simulink model "clarke"  (R2022b)
settings: Solver=VariableStepAuto  StartTime=0.0  StopTime=0.001  RelTol=1e-3
settings Model: Creator=15403  LastModifiedBy=15403

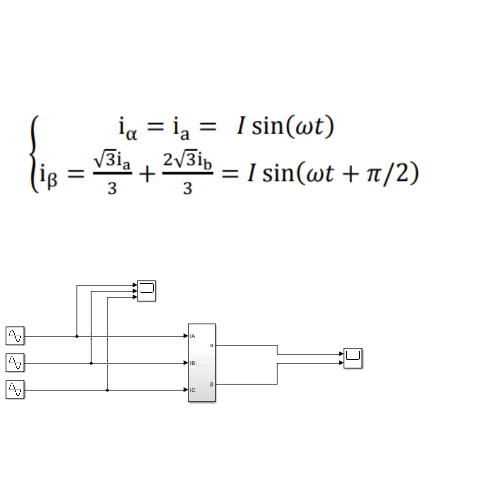
[thumbnail: Simulink's stored preview of the top-level diagram]
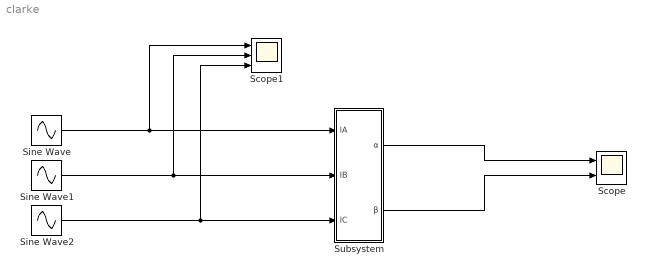
== system clarke ==
  Scope : Scope  NumInputPorts=2
  Scope1 : Scope  NumInputPorts=3
  Sine Wave : Sin  Amplitude=24/sqrt(3)  Frequency=2*pi*15000  SampleTime=0
  Sine Wave1 : Sin  Amplitude=24/sqrt(3)  Frequency=2*pi*15000  Phase=2*pi/3  SampleTime=0
  Sine Wave2 : Sin  Amplitude=24/sqrt(3)  Frequency=2*pi*15000  Phase=4*pi/3  SampleTime=0
  Subsystem : Subsystem
  wires:
  Sine Wave/1 -> Scope1/1, Subsystem/1(IA)
  Sine Wave1/1 -> Scope1/2, Subsystem/2(IB)
  Sine Wave2/1 -> Scope1/3, Subsystem/3(IC)
  Subsystem/1(α) -> Scope/1
  Subsystem/2(β) -> Scope/2

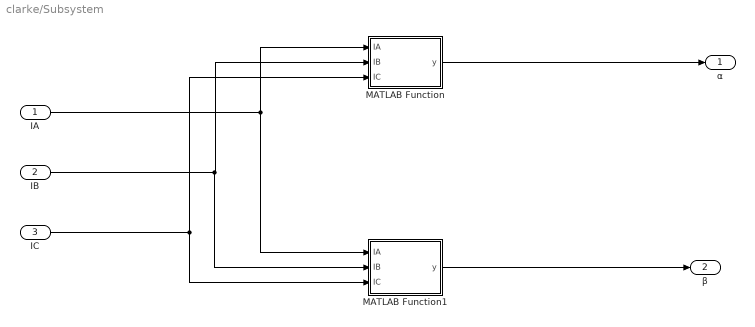
== system clarke/Subsystem ==
  IA : Inport
  IB : Inport  Port=2
  IC : Inport  Port=3
  MATLAB Function : MATLAB Function  TreatAsAtomicUnit=on
  MATLAB Function1 : MATLAB Function  TreatAsAtomicUnit=on
  α : Outport
  β : Outport  Port=2
  wires:
  MATLAB Function1/1(y) -> β/1
  MATLAB Function/1(y) -> α/1
  IA/1 -> MATLAB Function1/1(IA), MATLAB Function/1(IA)
  IB/1 -> MATLAB Function1/2(IB), MATLAB Function/2(IB)
  IC/1 -> MATLAB Function/3(IC), MATLAB Function1/3(IC)

== matlab function clarke/Subsystem/MATLAB Function1 ==
  data: IA input; y output; IB input; IC input
function y = fcn(IA, IB, IC)
%y = sqrt(3)/2 * IB - sqrt(3)/2 * IC;
y = (IB - IC) * cosd(30);

== matlab function clarke/Subsystem/MATLAB Function ==
  data: y output; IA input; IB input; IC input
function y = fcn(IA, IB, IC)
%y = IA - 1/2*IB-1/2*IC;
y = IA - (IB + IC) * cosd(60);
